simulink model "mWriteMask"  (R2021a)
settings: Solver=FixedStepAuto  StartTime=0.0  StopTime=inf  RelTol=1e-3  EnableMultiTasking=on
settings Model: SILPILModeSetting=veronly  ExtModeTrigDuration=2  Creator=angelo  LastModifiedBy=angelo
settings OptimizationCC: EnhancedBackFolding=on  PassReuseOutputArgsAs=Individual arguments  ZeroExternalMemoryAtStartup=off  ZeroInternalMemoryAtStartup=off  MaxStackSize=64  OptimizeBlockOrder=speed  DifferentSizesBufferReuse=on  OptimizationCustomize=off  EfficientTunableParamExpr=on
settings DebuggingCC: ParameterTunabilityLossMsg=error
settings HardwareCC: ProdBitPerInt=16  ProdBitPerPointer=16  ProdBitPerSizeT=16  ProdBitPerPtrDiffT=16  ProdLargestAtomicFloat=None  ProdWordSize=8  ProdHWDeviceType=Atmel->AVR
settings SFSimCC: MATLABDynamicMemAlloc=off
settings RTWCC: SystemTargetFile=ert.tlc  HardwareBoard=Arduino Mega 2560  TemplateMakefile=ert_default_tmf  Toolchain=Arduino AVR  BuildConfiguration=Faster Runs
settings CodeAppCC: ForceParamTrailComments=on  IgnoreCustomStorageClasses=off  OperatorAnnotations=on  SimulinkDataObjDesc=on  SFDataObjDesc=on  InsertBlockDesc=on
settings ERTTargetCC: SupportContinuousTime=on  SupportVariableSizeSignals=on  ExtModeStaticAllocSize=2048

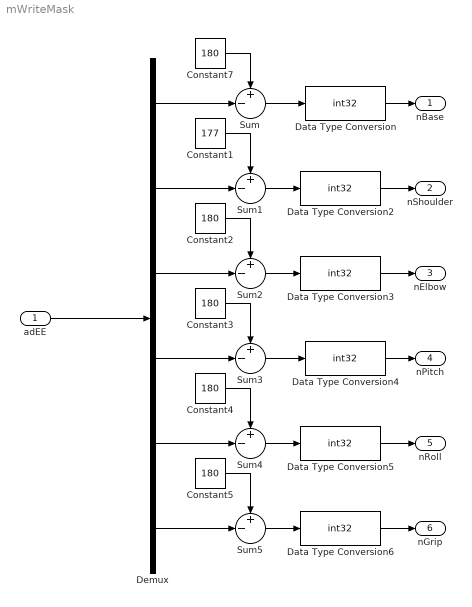
== system mWriteMask ==
  adEE : Inport
  Constant1 : Constant  Value=177
  Constant{2..5,7} (5 alike) : Constant  Value=180
  Data Type Conversion{,2..6} (6 alike) : DataTypeConversion  OutDataTypeStr=int32  RndMeth=Round
  Demux : Demux  Outputs=6
  Sum{,1..5} (6 alike) : Sum  Inputs=+-|
  nBase : Outport
  nShoulder : Outport  Port=2
  nElbow : Outport  Port=3
  nPitch : Outport  Port=4
  nRoll : Outport  Port=5
  nGrip : Outport  Port=6
  wires:
  Data Type Conversion4/1 -> nPitch/1
  Sum1/1 -> Data Type Conversion2/1
  Constant7/1 -> Sum/1
  Demux/6 -> Sum5/2
  Demux/1 -> Sum/2
  Data Type Conversion/1 -> nBase/1
  Demux/5 -> Sum4/2
  Sum3/1 -> Data Type Conversion4/1
  Sum2/1 -> Data Type Conversion3/1
  Data Type Conversion2/1 -> nShoulder/1
  adEE/1 -> Demux/1
  Constant2/1 -> Sum2/1
  Data Type Conversion5/1 -> nRoll/1
  Demux/3 -> Sum2/2
  Constant1/1 -> Sum1/1
  Data Type Conversion3/1 -> nElbow/1
  Constant3/1 -> Sum3/1
  Constant4/1 -> Sum4/1
  Constant5/1 -> Sum5/1
  Sum5/1 -> Data Type Conversion6/1
  Demux/2 -> Sum1/2
  Demux/4 -> Sum3/2
  Sum/1 -> Data Type Conversion/1
  Data Type Conversion6/1 -> nGrip/1
  Sum4/1 -> Data Type Conversion5/1
